simulink model "part7"  (R2014a)
settings: Solver=ode45  StartTime=0.0  StopTime=10.0  RelTol=1e-3
settings Model: Creator=SuperUser  LastModifiedBy=SuperUser

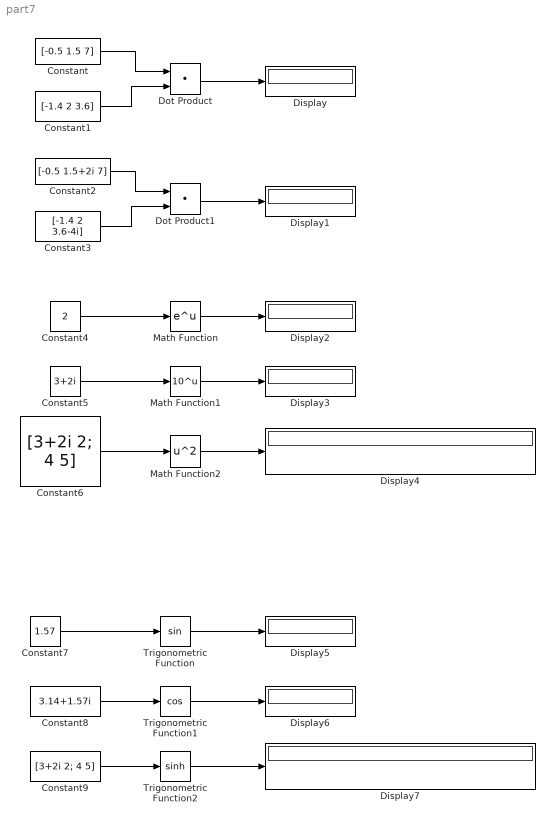
== system part7 ==
  Constant : Constant  Value=[-0.5 1.5 7]  VectorParams1D=off
  Constant1 : Constant  Value=[-1.4 2 3.6]
  Constant2 : Constant  Value=[-0.5 1.5+2i 7]  VectorParams1D=off
  Constant3 : Constant  Value=[-1.4 2 3.6-4i]
  Constant4 : Constant  Value=2
  Constant5 : Constant  Value=3+2i
  Constant6 : Constant  Value=[3+2i 2; 4 5]
  Constant7 : Constant  Value=1.57
  Constant8 : Constant  Value=3.14+1.57i
  Constant9 : Constant  Value=[3+2i 2; 4 5]
  Display{,1..7} (8 alike) : Display
  Dot Product : DotProduct  InputSameDT=on  OutDataTypeStr=Inherit: Inherit via internal rule
  Dot Product1 : DotProduct  InputSameDT=on  OutDataTypeStr=Inherit: Inherit via internal rule
  Math Function : Math  SaturateOnIntegerOverflow=on
  Math Function1 : Math  Operator=10^u  SaturateOnIntegerOverflow=on
  Math Function2 : Math  Operator=square  SaturateOnIntegerOverflow=on
  Trigonometric Function : Trigonometry
  Trigonometric Function1 : Trigonometry  Operator=cos
  Trigonometric Function2 : Trigonometry  Operator=sinh
  wires:
  Constant/1 -> Dot Product/1
  Constant1/1 -> Dot Product/2
  Dot Product/1 -> Display/1
  Constant2/1 -> Dot Product1/1
  Constant3/1 -> Dot Product1/2
  Dot Product1/1 -> Display1/1
  Constant4/1 -> Math Function/1
  Math Function/1 -> Display2/1
  Constant5/1 -> Math Function1/1
  Math Function1/1 -> Display3/1
  Constant6/1 -> Math Function2/1
  Math Function2/1 -> Display4/1
  Constant7/1 -> Trigonometric Function/1
  Trigonometric Function/1 -> Display5/1
  Constant8/1 -> Trigonometric Function1/1
  Trigonometric Function1/1 -> Display6/1
  Constant9/1 -> Trigonometric Function2/1
  Trigonometric Function2/1 -> Display7/1
